simulink model "heli"  (R2024b)
settings: Solver=VariableStepAuto  StartTime=0.0  StopTime=50.0  RelTol=1e-3
values from neighbouring files (symbols this model uses):
  A = [0      0      1       0 ... (first row only)    [HeliControl.m]    (also in heli.mat = [0 0 -1.263 0 0 0 0 0 1 0 -0.5437 0 ... (16 elements, 4x4)])
  B = [kp         0 ... (first row only)    [HeliControl.m]    (also in heli.mat = [0.035807  0; 0.035487  0; 0.0223  0; 0  -0.051391])
  C = [1 0 0 0 ... (first row only)    [HeliControl.m]    (also in heli.mat = [1  0  0  0; 0  1  0  0])
  K = Ksp(:,1:4)    [HeliControl.m]    (also in heli.mat = [34.813510404  38.1142478526  11.5999718061  16.4771259955; )
  Ki = -Ksp (:,5:6)    [HeliControl.m]    (also in heli.mat = [16.7968563908  18.7622888301; 16.9519622271  -25.0672997929)
  KiL = -Ksq (:,5:6)    [HeliControl.m]    (also in heli.mat = [18.4395474606  8.94379923323; 25.2968843496  -26.0774581028)
  KL = Ksq(:,1:4)    [HeliControl.m]    (also in heli.mat = [17.2717644019  13.5480013895  9.53777703233  3.91796069968;)
settings Model: Creator=nagel  LastModifiedBy=wilbe

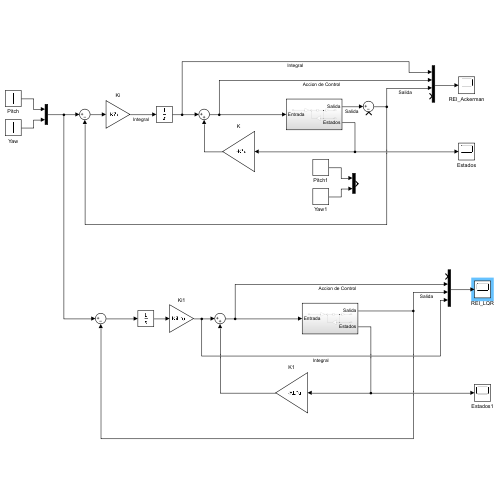
[thumbnail: Simulink's stored preview of the top-level diagram]
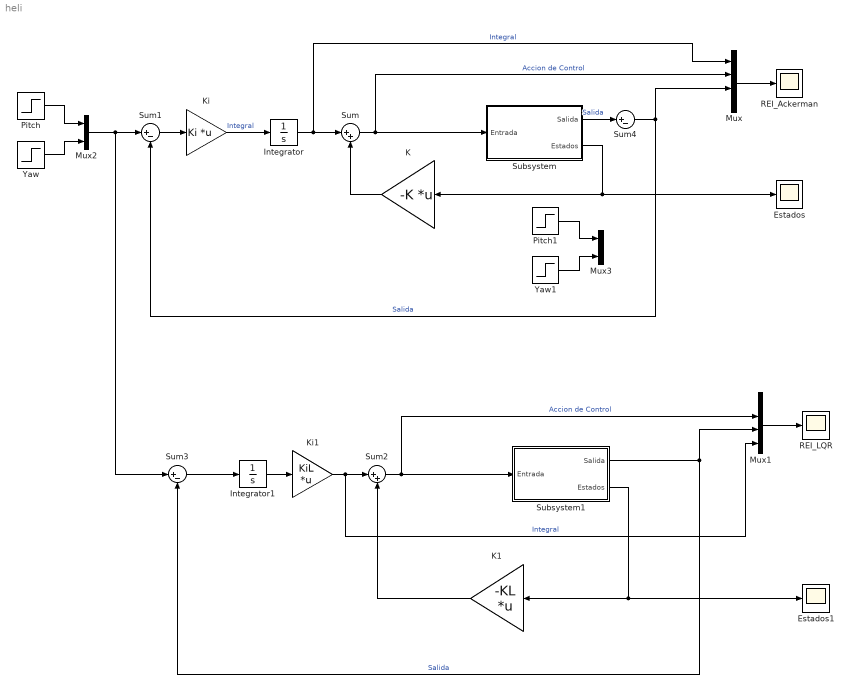
== system heli ==
  Estados : Scope
  Estados1 : Scope
  Integrator : Integrator
  Integrator1 : Integrator
  K : Gain  Gain=-K  Multiplication=Matrix(K*u)
  K1 : Gain  Gain=-KL  Multiplication=Matrix(K*u)
  Ki : Gain  Gain=Ki  Multiplication=Matrix(K*u)
  Ki1 : Gain  Gain=KiL  Multiplication=Matrix(K*u)
  Mux : Mux
  Mux1 : Mux
  Mux2 : Mux  Inputs=2
  Mux3 : Mux  Inputs=2
  Pitch : Step  Time=0  After=0.583  SampleTime=0.02
  Pitch1 : Step  Time=5  After=0.583  SampleTime=0.02
  REI_Ackerman : Scope
  REI_LQR : Scope
  Subsystem : Subsystem
  Subsystem1 : Subsystem
  Sum : Sum  Inputs=|++
  Sum1 : Sum  Inputs=|+-
  Sum2 : Sum  Inputs=|++
  Sum3 : Sum  Inputs=|+-
  Sum4 : Sum  Inputs=|+-
  Yaw : Step  Time=0  After=0  SampleTime=0.02
  Yaw1 : Step  Time=5  After=0.583  SampleTime=0
  wires:
  Subsystem/1(Salida) -> Sum4/1  "Salida"
  Subsystem/2(Estados) -> Estados/1, K/1
  Sum/1 -> Subsystem/1(Entrada), Mux/2  "Accion de Control"
  K/1 -> Sum/2
  Mux/1 -> REI_Ackerman/1
  Sum2/1 -> Subsystem1/1(Entrada), Mux1/2  "Accion de Control"
  Integrator1/1 -> Ki1/1
  K1/1 -> Sum2/2
  Sum3/1 -> Integrator1/1
  Mux1/1 -> REI_LQR/1
  Ki1/1 -> Mux1/4, Sum2/1  "Integral"
  Subsystem1/2(Estados) -> K1/1, Estados1/1
  Subsystem1/1(Salida) -> Sum3/2, Mux1/3  "Salida"
  Pitch/1 -> Mux2/1
  Yaw/1 -> Mux2/2
  Mux2/1 -> Sum3/1, Sum1/1
  Sum1/1 -> Ki/1
  Ki/1 -> Integrator/1  "Integral"
  Yaw1/1 -> Mux3/2
  Pitch1/1 -> Mux3/1
  Sum4/1 -> Mux/3, Sum1/2  "Salida"
  Integrator/1 -> Mux/1, Sum/1  "Integral"

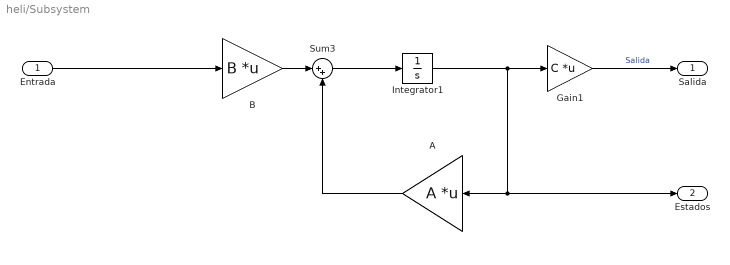
== system heli/Subsystem ==
  Entrada : Inport
  A : Gain  Gain=A  Multiplication=Matrix(K*u)
  B : Gain  Gain=B  Multiplication=Matrix(K*u)
  Gain1 : Gain  Gain=C  Multiplication=Matrix(K*u)
  Integrator1 : Integrator
  Sum3 : Sum  Inputs=|++
  Salida : Outport
  Estados : Outport  Port=2
  wires:
  Sum3/1 -> Integrator1/1
  B/1 -> Sum3/1
  A/1 -> Sum3/2
  Gain1/1 -> Salida/1  "Salida"
  Integrator1/1 -> A/1, Estados/1, Gain1/1
  Entrada/1 -> B/1

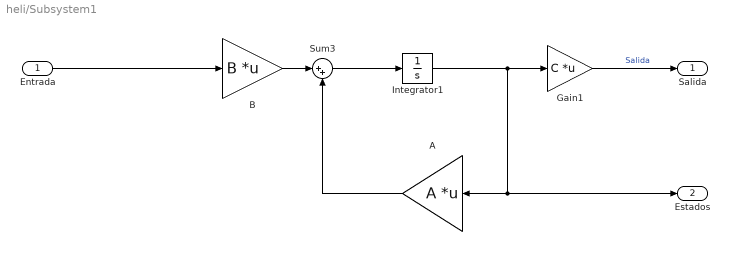
== system heli/Subsystem1 ==
  Entrada : Inport
  A : Gain  Gain=A  Multiplication=Matrix(K*u)
  B : Gain  Gain=B  Multiplication=Matrix(K*u)
  Gain1 : Gain  Gain=C  Multiplication=Matrix(K*u)
  Integrator1 : Integrator
  Sum3 : Sum  Inputs=|++
  Salida : Outport
  Estados : Outport  Port=2
  wires:
  Sum3/1 -> Integrator1/1
  B/1 -> Sum3/1
  A/1 -> Sum3/2
  Gain1/1 -> Salida/1  "Salida"
  Integrator1/1 -> A/1, Estados/1, Gain1/1
  Entrada/1 -> B/1
